simulink model "Copy_of_PDUSTM32"  (R2024b)
settings: Solver=FixedStepDiscrete  StartTime=0.0  StopTime=1  FixedStep=0.001  RelTol=1e-3  EnableMultiTasking=on
libraries: stm32blockslib x32, stm32f4xxblockslib x14, canmsglib x7, simulink x3, stm32h7xxblockslib x1
(part 3 of 3)

== matlab function Copy_of_PDUSTM32/CAN TX2/MATLAB Function2 ==
  settings: updateMethod=DISCRETE  sampleTime=.001
  data: WriteInstruction output; ID input uint32; CANVector output uint8; Length input uint8; Data input uint8; RTS input; RTSByte output; period input; offset input; MCPInitialized input
function [WriteInstruction, CANVector, RTSByte] = ConvertToVector(ID, Length, Data, RTS, period, offset, MCPInitialized)
%#codegen
persistent count;
if isempty(count)
    count = uint16(0);
end

if MCPInitialized
    if count == uint16(offset)
        id_u16 = uint16(ID);
        CANVector = zeros(1,13,'uint8');
        CANVector(1) = uint8(bitshift(id_u16, -3));
        CANVector(2) = uint8(bitshift(bitand(id_u16, uint16(7)), 5));
        CANVector(3) = uint8(0);
        CANVector(4) = uint8(0);
        CANVector(5) = bitand(uint8(Length), uint8(15));
        for i = 1:8
            CANVector(5+i) = uint8(Data(i));
        end
        RTSByte = uint8(RTS);
        WriteInstruction = uint8(0x02);
    else
        CANVector = zeros(1,13,'uint8');
        RTSByte = uint8(0x03);
        WriteInstruction = uint8(0x03);
    end

    count = count + uint16(1);
    if count >= uint16(period)
        count = uint16(0);
    end
else
    CANVector = zeros(1,13,'uint8');
    RTSByte = uint8(0x03);
    WriteInstruction = uint8(0x03);
    % don't increment count while MCP not ready
end

== matlab function Copy_of_PDUSTM32/ADC121S021 1/MATLAB Function ==
  data: Counts input uint8; Voltage output; VA input double; raww output
function [Voltage, raww]= ConvertToVoltage(Counts, VA)
    raw = uint16(Counts(1)) * 256 + uint16(Counts(2));
    counts = double(bitshift(raw, -1) & uint16(4095));
    Voltage = double(counts * (VA / 4095.0));
    raww = Counts(1);
end

== matlab function Copy_of_PDUSTM32/CAN Rx/CAN RX2/Enabled Subsystem/MATLAB Function7 ==
  data: RxBytes input uint8 size=15; Message output Bus: CANMessage
function Message = DecodeCANMsg(RxBytes)
%#codegen
% RxBytes is uint8(1x15); bytes 1-2 are don't-care (command echo + one turnaround byte)
SIDH = RxBytes(3);
SIDL = RxBytes(4);
EID8 = RxBytes(5);
EID0 = RxBytes(6);
DLC  = RxBytes(7);

Message.ID       = uint32(bitor(uint32(bitshift(uint32(SIDH), 3)), ...
                        uint32(bitshift(uint32(SIDL), -5))));
Message.Extended = false;
Message.Remote   = false;
Message.Error    = false;
Message.Length   = double(bitand(DLC, uint8(15)));
Message.Data     = RxBytes(8:15);

== matlab function Copy_of_PDUSTM32/CAN TX5/MATLAB Function2 ==
  settings: updateMethod=DISCRETE  sampleTime=.001
  data: WriteInstruction output; ID input uint32; CANVector output uint8; Length input uint8; Data input uint8; RTS input; RTSByte output; period input; offset input; MCPInitialized input
function [WriteInstruction, CANVector, RTSByte] = ConvertToVector(ID, Length, Data, RTS, period, offset, MCPInitialized)
%#codegen
persistent count;
if isempty(count)
    count = uint16(0);
end

if MCPInitialized
    if count == uint16(offset)
        id_u16 = uint16(ID);
        CANVector = zeros(1,13,'uint8');
        CANVector(1) = uint8(bitshift(id_u16, -3));
        CANVector(2) = uint8(bitshift(bitand(id_u16, uint16(7)), 5));
        CANVector(3) = uint8(0);
        CANVector(4) = uint8(0);
        CANVector(5) = bitand(uint8(Length), uint8(15));
        for i = 1:8
            CANVector(5+i) = uint8(Data(i));
        end
        RTSByte = uint8(RTS);
        WriteInstruction = uint8(0x02);
    else
        CANVector = zeros(1,13,'uint8');
        RTSByte = uint8(0x03);
        WriteInstruction = uint8(0x03);
    end

    count = count + uint16(1);
    if count >= uint16(period)
        count = uint16(0);
    end
else
    CANVector = zeros(1,13,'uint8');
    RTSByte = uint8(0x03);
    WriteInstruction = uint8(0x03);
    % don't increment count while MCP not ready
end

== matlab function Copy_of_PDUSTM32/ADC121S021 2/MATLAB Function ==
  data: Counts input uint8; Voltage output double; VA input double
function Voltage = ConvertToVoltage(Counts, VA)
    raw = uint16(Counts(1)) * 256 + uint16(Counts(2));
    counts = double(bitshift(raw, -1) & uint16(4095));
    Voltage = double(counts * (VA / 4095.0));
end

== matlab function Copy_of_PDUSTM32/ADC121S021 3/MATLAB Function ==
  data: Counts input uint8; Voltage output double; VA input double
function Voltage = ConvertToVoltage(Counts, VA)
    raw = uint16(Counts(1)) * 256 + uint16(Counts(2));
    counts = double(bitshift(raw, -1) & uint16(4095));
    Voltage = double(counts * (VA / 4095.0));
end

== matlab function Copy_of_PDUSTM32/ADC121S021 4/MATLAB Function ==
  data: Counts input uint8; Voltage output double; VA input double
function Voltage = ConvertToVoltage(Counts, VA)
    raw = uint16(Counts(1)) * 256 + uint16(Counts(2));
    counts = double(bitshift(raw, -1) & uint16(4095));
    Voltage = double(counts * (VA / 4095.0));
end

== matlab function Copy_of_PDUSTM32/CAN TX6/MATLAB Function2 ==
  settings: updateMethod=DISCRETE  sampleTime=.001
  data: WriteInstruction output; ID input uint32; CANVector output uint8; Length input uint8; Data input uint8; RTS input; RTSByte output; period input; offset input; MCPInitialized input
function [WriteInstruction, CANVector, RTSByte] = ConvertToVector(ID, Length, Data, RTS, period, offset, MCPInitialized)
%#codegen
persistent count;
if isempty(count)
    count = uint16(0);
end

if MCPInitialized
    if count == uint16(offset)
        id_u16 = uint16(ID);
        CANVector = zeros(1,13,'uint8');
        CANVector(1) = uint8(bitshift(id_u16, -3));
        CANVector(2) = uint8(bitshift(bitand(id_u16, uint16(7)), 5));
        CANVector(3) = uint8(0);
        CANVector(4) = uint8(0);
        CANVector(5) = bitand(uint8(Length), uint8(15));
        for i = 1:8
            CANVector(5+i) = uint8(Data(i));
        end
        RTSByte = uint8(RTS);
        WriteInstruction = uint8(0x02);
    else
        CANVector = zeros(1,13,'uint8');
        RTSByte = uint8(0x03);
        WriteInstruction = uint8(0x03);
    end

    count = count + uint16(1);
    if count >= uint16(period)
        count = uint16(0);
    end
else
    CANVector = zeros(1,13,'uint8');
    RTSByte = uint8(0x03);
    WriteInstruction = uint8(0x03);
    % don't increment count while MCP not ready
end

== matlab function Copy_of_PDUSTM32/MATLAB Function2 ==
  settings: updateMethod=DISCRETE  sampleTime=.001
  data: WriteInstruction output; ID input uint32; CANVector output uint8; Length input uint8; Data input uint8; RTS input; RTSByte output; period input; offset input; MCPInitialized input
function [WriteInstruction, CANVector, RTSByte] = ConvertToVector(ID, Length, Data, RTS, period, offset, MCPInitialized)
%#codegen
% Inputs (N = 3 messages):
%   ID      : 1x3  (11-bit standard IDs)
%   Length  : 1x3  (DLC, 0-8)
%   Data    : 3x8  (row i = data bytes of message i)
%   RTS     : 1x3  (RTS instruction byte for each message; for TXB0 this is 0x81)
%   period  : 1x3  (in steps)
%   offset  : 1x3  (in steps)
% Outputs, row/element i belongs to message i:
%   WriteInstruction : 1x3  (0x02 = write, 0x03 = no-op sentinel as in your original)
%   CANVector        : 3x13 (SIDH, SIDL, EID8, EID0, DLC, D0..D7)
%   RTSByte          : 1x3

N = 3;

persistent count;
if isempty(count)
    count = zeros(1, N, 'uint16');
end

WriteInstruction = repmat(uint8(0x03), 1, N);
RTSByte          = repmat(uint8(0x03), 1, N);
CANVector        = zeros(N, 13, 'uint8');

if MCPInitialized
    for m = 1:N
        if count(m) == uint16(offset(m))
            id_u16 = uint16(ID(m));
            CANVector(m,1) = uint8(bitshift(id_u16, -3));
            CANVector(m,2) = uint8(bitshift(bitand(id_u16, uint16(7)), 5));
            CANVector(m,3) = uint8(0);
            CANVector(m,4) = uint8(0);
            CANVector(m,5) = bitand(uint8(Length(m)), uint8(15));
            for i = 1:8
                CANVector(m,5+i) = uint8(Data(m,i));
            end
            RTSByte(m)          = uint8(RTS(m));
            WriteInstruction(m) = uint8(0x02);
        end

        count(m) = count(m) + uint16(1);
        if count(m) >= uint16(period(m))
            count(m) = uint16(0);
        end
    end
end
% counts don't increment while the MCP isn't initialized
end
